simulink model "Simulation2"  (R2024b)
settings: Solver=VariableStepAuto  StartTime=0.0  StopTime=30  RelTol=1e-3
libraries: vrlib x1
settings Model: SimulationMode=accelerator  PacingRate=0.980000  Creator=alvinisac  LastModifiedBy=alvinisac

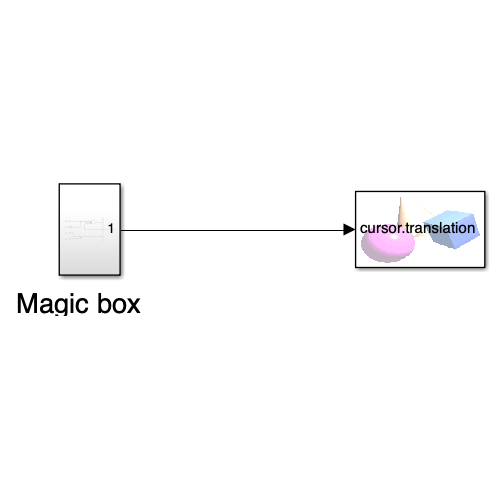
[thumbnail: Simulink's stored preview of the top-level diagram]
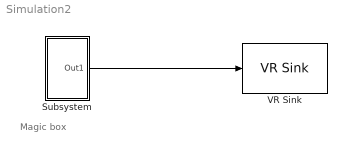
== system Simulation2 ==
  note: Magic box
  Subsystem : Subsystem
  VR Sink : vrlib/VR Sink  InstantiateOnLoad=on  SampleTime=0.1  ViewEnable=on  RemoteChange=off  RemoteView=off  FieldsWritten=cursor.translation.3.1.1.double  WorldFileName=8_palline_color.wrl  AutoView=off  VideoDimensions=[]  AllowVariableSize=off  FigureProperties="{'Position', 'Name', 'Viewpoint', 'CameraBound', 'CameraDirection', 'CameraPosition', 'CameraUpVector', 'ZoomFactor', 'Antialiasing', 'Headlight', 'Lighting', 'Sound', 'StatusBar', 'Stereo3D', 'Stereo3DCameraOffset', 'Stereo3DHIT', 'ToolBar', 'Textures', 'Transparency', 'Triad', 'Wireframe', 'NavZones', 'NavMode', 'NavSpeed', 'CaptureFileFormat', 'CaptureFileName', 'Record2DCompressMethod', 'Record2DCompressQuality', 'Record2D', 'Record2DFileName', 'Record2DFPS', 'NavPanel'; [-6.8300000000000000e+02   1.1100000000000000e+02   6.7600000000000000e+02   7.2100000000000000e+02], '', '_untitled_1', 'on', [0.0000000000000000e+00   0.0000000000000000e+00  -1.0000000000000000e+00], [0.0000000000000000e+00   0.0000000000000000e+00   0.0000000000000000e+00], [0.0000000000000000e+00   1.0000000000000000e+00   0.0000000000000000e+00], [1.0000000000000000e+00], 'on', 'on', 'on', 'on', 'on', 'off', [1.0000000149011612e-01], [0.0000000000000000e+00], 'on', 'on', 'on', 'none', 'off', 'off', 'fly', 'normal', 'tif', '%f_anim_%n.tif', 'auto', [7.5000000000000000e+01], 'off', '%f_anim_%n.avi', 'auto', 'halfbar'}"
  wires:
  Subsystem/1(Out1) -> VR Sink/1

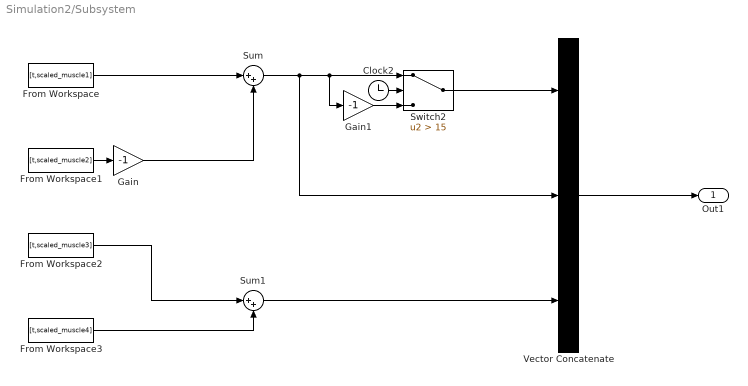
== system Simulation2/Subsystem ==
  Clock2 : Clock
  From Workspace : FromWorkspace  VariableName=[t,scaled_muscle1]
  From Workspace1 : FromWorkspace  VariableName=[t,scaled_muscle2]
  From Workspace2 : FromWorkspace  VariableName=[t,scaled_muscle3]
  From Workspace3 : FromWorkspace  VariableName=[t,scaled_muscle4]
  Gain : Gain  Gain=-1
  Gain1 : Gain  Gain=-1
  Sum : Sum  Inputs=|++
  Sum1 : Sum  Inputs=|++
  Switch2 : Switch  Criteria=u2 > Threshold  Threshold=15  SaturateOnIntegerOverflow=off  InputSameDT=off
  Vector Concatenate : Concatenate  NumInputs=3
  Out1 : Outport
  wires:
  From Workspace3/1 -> Sum1/2
  Vector Concatenate/1 -> Out1/1
  From Workspace2/1 -> Sum1/1
  Switch2/1 -> Vector Concatenate/1
  Clock2/1 -> Switch2/2
  From Workspace1/1 -> Gain/1
  Gain/1 -> Sum/2
  Gain1/1 -> Switch2/3
  Sum1/1 -> Vector Concatenate/3
  Sum/1 -> Switch2/1, Gain1/1, Vector Concatenate/2
  From Workspace/1 -> Sum/1
